simulink subsystem "EoM_Euler5DoF"  (R2024b)
settings: Solver=VariableStepAuto  StartTime=0.0  StopTime=10.0  RelTol=1e-3
values from neighbouring files (symbols this model uses):
  vehicle = load("Astra2").vehicle    [TrajOptimizer5DoF_test_script.m]
undefined symbols (not defined in the file or in its folder): com_error, inertia_error, mass_error
settings Model: Creator=thatf  LastModifiedBy=thatf

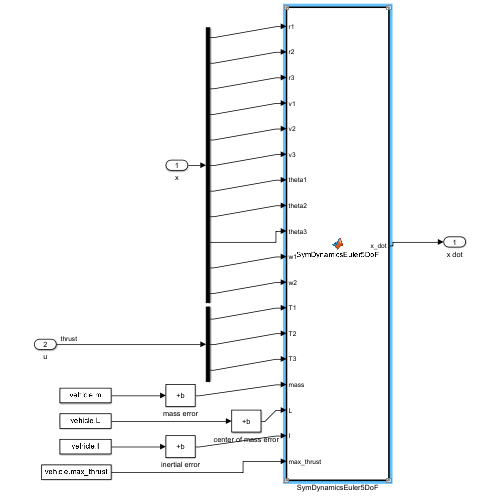
[thumbnail: Simulink's stored preview of the top-level diagram]
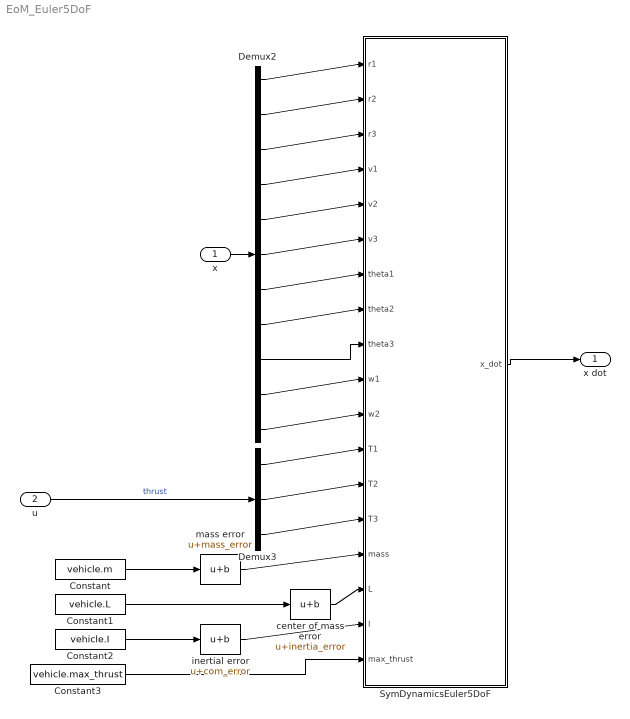
== system EoM_Euler5DoF ==
  x : Inport
  u : Inport  Port=2
  Constant : Constant  Value=vehicle.m
  Constant1 : Constant  Value=vehicle.L
  Constant2 : Constant  Value=vehicle.I
  Constant3 : Constant  Value=vehicle.max_thrust
  Demux2 : Demux  Outputs=11
  Demux3 : Demux  Outputs=3
  SymDynamicsEuler5DoF : MATLAB Function  TreatAsAtomicUnit=on
  center of mass error : Bias  Bias=inertia_error  SaturateOnIntegerOverflow=off
  inertial error : Bias  Bias=com_error  SaturateOnIntegerOverflow=off
  mass error : Bias  Bias=mass_error  SaturateOnIntegerOverflow=off
  x dot : Outport
  wires:
  x/1 -> Demux2/1
  Constant1/1 -> center of mass error/1
  Constant2/1 -> inertial error/1
  SymDynamicsEuler5DoF/1(x_dot) -> x dot/1
  u/1 -> Demux3/1  "thrust"
  mass error/1 -> SymDynamicsEuler5DoF/15(mass)
  Constant/1 -> mass error/1
  center of mass error/1 -> SymDynamicsEuler5DoF/16(L)
  inertial error/1 -> SymDynamicsEuler5DoF/17(I)
  Demux3/1 -> SymDynamicsEuler5DoF/12(T1)
  Demux2/11 -> SymDynamicsEuler5DoF/11(w2)
  Demux2/10 -> SymDynamicsEuler5DoF/10(w1)
  Demux2/9 -> SymDynamicsEuler5DoF/9(theta3)
  Demux2/8 -> SymDynamicsEuler5DoF/8(theta2)
  Demux2/1 -> SymDynamicsEuler5DoF/1(r1)
  Demux2/2 -> SymDynamicsEuler5DoF/2(r2)
  Demux2/3 -> SymDynamicsEuler5DoF/3(r3)
  Demux2/4 -> SymDynamicsEuler5DoF/4(v1)
  Demux2/5 -> SymDynamicsEuler5DoF/5(v2)
  Demux2/6 -> SymDynamicsEuler5DoF/6(v3)
  Demux2/7 -> SymDynamicsEuler5DoF/7(theta1)
  Demux3/2 -> SymDynamicsEuler5DoF/13(T2)
  Demux3/3 -> SymDynamicsEuler5DoF/14(T3)
  Constant3/1 -> SymDynamicsEuler5DoF/18(max_thrust)

== matlab function EoM_Euler5DoF/SymDynamicsEuler5DoF ==
  data: r1 input; x_dot output; r2 input; r3 input; v1 input; v2 input; v3 input; theta1 input; theta2 input; theta3 input; w1 input; w2 input; T1 input; T2 input; T3 input; mass input; L input; I input; max_thrust input
function x_dot = SymDynamicsEuler5DoF(r1,r2,r3,v1,v2,v3,theta1,theta2,theta3,w1,w2,T1,T2,T3,mass,L,I,max_thrust)
%#codegen

%    This function was generated by the Symbolic Math Toolbox version 24.2.
%    03-Jan-2025 22:18:37

% r1 = complex(r1);  % if required to enforce complex operations
% r2 = complex(r2);  % if required to enforce complex operations
% r3 = complex(r3);  % if required to enforce complex operations
% v1 = complex(v1);  % if required to enforce complex operations
% v2 = complex(v2);  % if required to enforce complex operations
% v3 = complex(v3);  % if required to enforce complex operations
% theta1 = complex(theta1);  % if required to enforce complex operations
% theta2 = complex(theta2);  % if required to enforce complex operations
% theta3 = complex(theta3);  % if required to enforce complex operations
% w1 = complex(w1);  % if required to enforce complex operations
% w2 = complex(w2);  % if required to enforce complex operations
% T1 = complex(T1);  % if required to enforce complex operations
% T2 = complex(T2);  % if required to enforce complex operations
% T3 = complex(T3);  % if required to enforce complex operations
% mass = complex(mass);  % if required to enforce complex operations
% L = complex(L);  % if required to enforce complex operations
% I = complex(I);  % if required to enforce complex operations
% max_thrust = complex(max_thrust);  % if required to enforce complex operations
t2 = cos(theta1);
t3 = cos(theta2);
t4 = cos(theta3);
t5 = sin(theta1);
t6 = sin(theta2);
t7 = sin(theta3);
t8 = 1.0./I;
t9 = 1.0./mass;
t10 = 1.0./t6;
x_dot = [v1;v2;v3;t9.*(T1.*max_thrust.*t3+T3.*max_thrust.*t4.*t6+T2.*max_thrust.*t6.*t7);t9.*(T2.*max_thrust.*(t2.*t4-t3.*t5.*t7)-T3.*max_thrust.*(t2.*t7+t3.*t4.*t5)+T1.*max_thrust.*t5.*t6);-t9.*(-T2.*max_thrust.*(t4.*t5+t2.*t3.*t7)+T3.*max_thrust.*(t5.*t7-t2.*t3.*t4)+T1.*max_thrust.*t2.*t6)-9.81e+2./1.0e+2;t4.*t10.*w2+t7.*t10.*w1;t4.*w1-t7.*w2;-t3.*t4.*t10.*w2-t3.*t7.*t10.*w1;L.*T3.*max_thrust.*t8;-L.*T2.*max_thrust.*t8];
end
